simulink library "library"  (R2023b)
settings: Solver=VariableStepAuto  StartTime=0.0  StopTime=10.0  RelTol=1e-3
undefined symbols (not defined in the file or in its folder): DiscIntNeverNeededParam, mmc
libraries: $bdroot x3, spsVoltageMeasurementLib x3, spsControlledVoltageSourceLib x3, eeDiscretePi x2, spsFullBridgeMMCLib x1, simulink x1
settings Model: Creator=ma1155716  LastModifiedBy=ma1155716

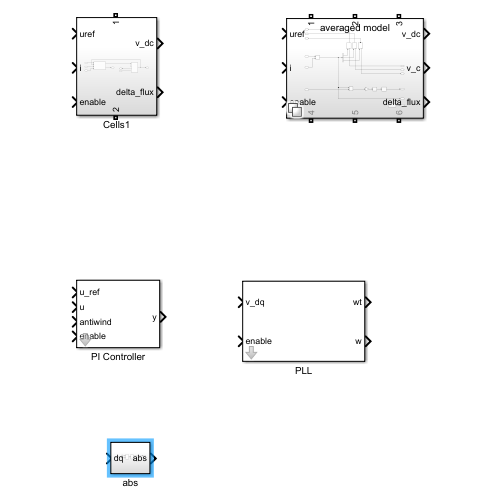
[thumbnail: Simulink's stored preview of the top-level diagram]
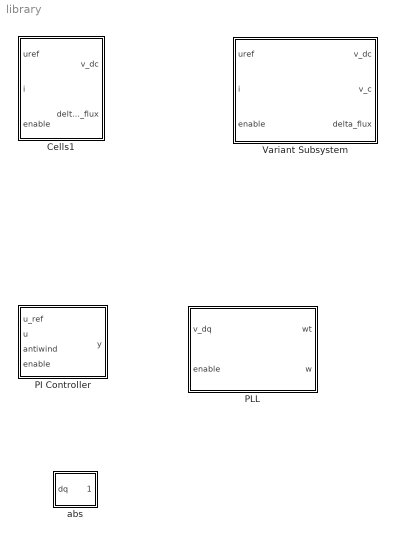
== system library ==
  Cells1 : Subsystem
      settings: PortSchema="{\"entries\":[{\"content\":{\"sides\":[{\"content\":{\"connectorIds\":[\"In1\",\"In2\",\"In3\"]},\"type\":\"ConnectorPlacement.EquallySpacedRectSide\",\"uuid\":\"5601622e-70e0-44e7-973e-d59d180f15ed\"},{\"content\":{\"connectorIds\":[\"Out1\",\"Out2\"],\"side\":\"RIGHT\"},\"type\":\"ConnectorPlacement.EquallySpacedRectSide\",\"uuid\":\"4beaff91-e32f-480b-a73b-58099df36fbd\"},{\"content\":{\"connectorIds\":[\"LConn1\"],\"side\":\"TOP\"},\"type\":\"ConnectorPlacement.EquallySpacedRectSide\",\"uuid\":\"32571f3d-d835-4e58-b20d-9f53f86bf78d\"},{\"content\":{\"connectorIds\":[\"RConn1\"],\"side\":\"BOTTOM\"},\"type\":\"ConnectorPlacement.EquallySpacedRectSide\",\"uuid\":\"b1b232fc-3b26-4ea5-8985-03b3a1c4d3e8\"}]},\"type\":\"ConnectorPlacement.EquallySpacedConnector\",\"uuid\":\"974b71ee-efdc-4c08-8e6f-7a03276fde15\"}],\"packageUris\":[\"http://schema.mathworks.com/mf0/Connector/R2020b\"],\"version\":\"1.0\"}"
  PI Controller : Subsystem  VariantControl=overcurr_ctrl.sel==1  mask{kp=0, ti=0, Kaw=1}
      mask prompts: kp "Proportional gain"; ti "Time constant"; Kaw "Anti windup gain"
  PLL : Subsystem  mask{kp=0, ti=0, w0=0, wn=0}
      mask prompts: kp "Proportional gain"; ti "Time constant"; w0 "Initial angular frequency"; wn "Nominal angular frequency"
  Variant Subsystem : Subsystem  Variant=on
      settings: PortSchema="{\"entries\":[{\"content\":{\"sides\":[{\"content\":{\"connectorIds\":[\"In1\",\"In2\",\"In3\"]},\"type\":\"ConnectorPlacement.EquallySpacedRectSide\",\"uuid\":\"07cc1b48-4eec-48c8-b7e1-ba85327af049\"},{\"content\":{\"connectorIds\":[\"Out1\",\"Out2\",\"Out3\"],\"side\":\"RIGHT\"},\"type\":\"ConnectorPlacement.EquallySpacedRectSide\",\"uuid\":\"e630ccd2-bced-4562-b965-5ba67d1cb520\"},{\"content\":{\"connectorIds\":[\"LConn1\",\"LConn2\",\"LConn3\"],\"side\":\"TOP\"},\"type\":\"ConnectorPlacement.EquallySpacedRectSide\",\"uuid\":\"f7ee33a5-0b9e-482c-ae72-b6ca50f6d328\"},{\"content\":{\"connectorIds\":[\"RConn1\",\"RConn2\",\"RConn3\"],\"side\":\"BOTTOM\"},\"type\":\"ConnectorPlacement.EquallySpacedRectSide\",\"uuid\":\"76c11136-f7c0-446b-9aed-353e2cf8a045\"}]},\"type\":\"ConnectorPlacement.EquallySpacedConnector\",\"uuid\":\"ad2af07b-650a-4f66-848d-c3c749fafa1e\"}],\"packageUris\":[\"http://schema.mathworks.com/mf0/Connector/R2020b\"],\"version\":\"1.0\"}"
  abs : Subsystem

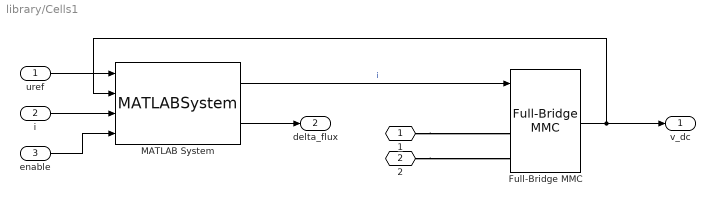
== system library/Cells1 ==
  uref : Inport
  i : Inport  Port=2
  enable : Inport  Port=3
  Full-Bridge MMC : spsFullBridgeMMCLib/Full-Bridge MMC  ModelType=Switching devices  n=mmc.cell.n  C=mmc.cell.c_dc  Vc_Initial=mmc.cell.v_dc  Ron=1e-3  Rs=1e6  Cs=inf  Ron_Diode=1e-3  Rs_Diode=1e6  Cs_Diode=inf  Vf_Diode=1e-3  Rs_CurrentSource=inf  Ts=10e-6
      settings: LibrarySourceBlock=sps_lib/Power Electronics/Full-Bridge MMC
  MATLAB System : MATLABSystem  System=CellSelector  ts=[1e-6]  f_carr=[3*50]  n_cells=[mmc.cell.n]  SimulateUsing=Code generation
      mask Type: CellSelector
      mask Display:
      | disp('CellSelector');
      | port_label('input',1,'v_ref');
      | port_label('input',2,'v_dc');
      | port_label('input',3,'i');
      | port_label('input',4,'enable');
      | port_label('output',1,'g');
      | port_label('output',2,'delta_flux');
  1 : PMIOPort  Side=Left
  2 : PMIOPort  Port=2  Side=Right
  v_dc : Outport
  delta_flux : Outport  Port=2
  wires:
  i/1 -> MATLAB System/3
  MATLAB System/2 -> delta_flux/1
  MATLAB System/1 -> Full-Bridge MMC/1  "i"
  uref/1 -> MATLAB System/1
  Full-Bridge MMC/1 -> MATLAB System/2, v_dc/1
  enable/1 -> MATLAB System/4
  connections:
  1/RConn1 -- Full-Bridge MMC/LConn1
  2/RConn1 -- Full-Bridge MMC/LConn2

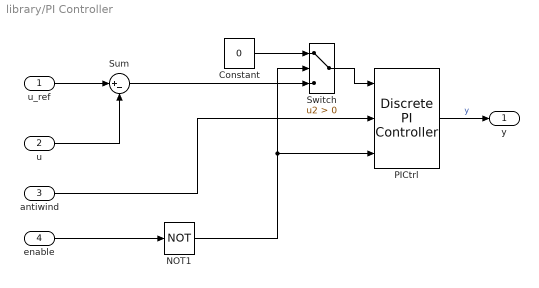
== system library/PI Controller ==
  u_ref : Inport
  u : Inport  Port=2
  antiwind : Inport  Port=3
  enable : Inport  Port=4
  Constant : Constant  Value=0
  NOT1 : Logic  Operator=NOT  IconShape=distinctive  AllPortsSameDT=off  OutDataTypeStr=boolean
  PICtrl : eeDiscretePi/Discrete PI Controller  Kp=kp  Ki=kp/ti  Kaw=Kaw  x0=0  Ts=-1
      settings: LibrarySourceBlock=ee_sl_lib/General Control/Discrete PI Controller
  Sum : Sum  Inputs=|+-
  Switch : Switch  Criteria=u2 > Threshold  SaturateOnIntegerOverflow=off  InputSameDT=off
  y : Outport
  wires:
  u_ref/1 -> Sum/1
  u/1 -> Sum/2
  NOT1/1 -> Switch/2, PICtrl/3
  enable/1 -> NOT1/1
  PICtrl/1 -> y/1  "y"
  antiwind/1 -> PICtrl/2
  Constant/1 -> Switch/1
  Switch/1 -> PICtrl/1
  Sum/1 -> Switch/3

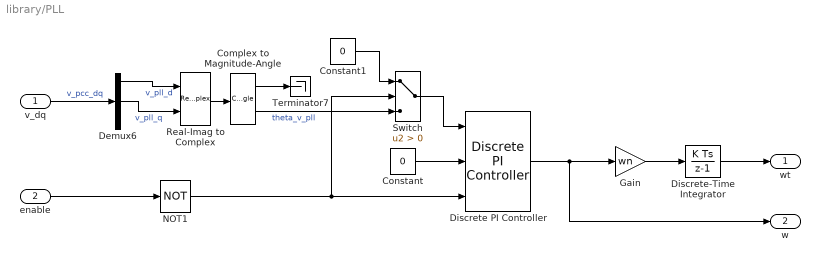
== system library/PLL ==
  v_dq : Inport
  enable : Inport  Port=2
  Complex to Magnitude-Angle : ComplexToMagnitudeAngle
  Constant : Constant  Value=0
  Constant1 : Constant  Value=0
  Demux6 : Demux  Outputs=3
  Discrete PI Controller : eeDiscretePi/Discrete PI Controller  Kp=kp  Ki=ti  Kaw=1  x0=w0  Ts=-1
      settings: LibrarySourceBlock=ee_sl_lib/General Control/Discrete PI Controller
  Discrete-Time Integrator : DiscreteIntegrator  gainval=1  SampleTime=-1  ICPrevOutput=DiscIntNeverNeededParam  ICPrevScaledInput=DiscIntNeverNeededParam
  Gain : Gain  Gain=wn
  NOT1 : Logic  Operator=NOT  IconShape=distinctive  AllPortsSameDT=off  OutDataTypeStr=boolean
  Real-Imag to Complex : RealImagToComplex
  Switch : Switch  Criteria=u2 > Threshold  SaturateOnIntegerOverflow=off  InputSameDT=off
  Terminator7 : Terminator
  wt : Outport
  w : Outport  Port=2
  wires:
  v_dq/1 -> Demux6/1  "v_pcc_dq"
  Complex to Magnitude-Angle/1 -> Terminator7/1
  Demux6/2 -> Real-Imag to Complex/2  "v_pll_q"
  Complex to Magnitude-Angle/2 -> Switch/3  "theta_v_pll"
  Real-Imag to Complex/1 -> Complex to Magnitude-Angle/1
  Demux6/1 -> Real-Imag to Complex/1  "v_pll_d"
  Constant/1 -> Discrete PI Controller/2
  Discrete PI Controller/1 -> w/1, Gain/1
  Discrete-Time Integrator/1 -> wt/1
  NOT1/1 -> Switch/2, Discrete PI Controller/3
  enable/1 -> NOT1/1
  Switch/1 -> Discrete PI Controller/1
  Constant1/1 -> Switch/1
  Gain/1 -> Discrete-Time Integrator/1

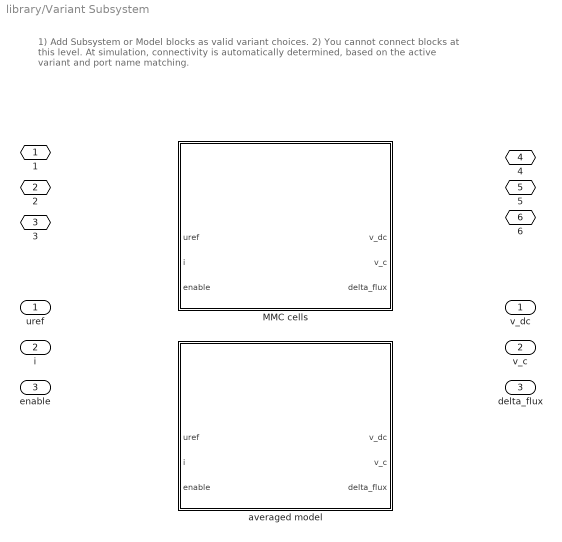
== system library/Variant Subsystem ==
  note: 1) Add Subsystem or Model blocks as valid variant choices.
      | 2) You cannot connect blocks at this level. At simulation, connectivity is automatically
      | determined, based on the active variant and port name matching.
  uref : Inport
  i : Inport  Port=2
  enable : Inport  Port=3
  MMC cells : Subsystem  VariantControl=ctrl.cell.sel==0
      settings: PortSchema="{\"entries\":[{\"content\":{\"sides\":[{\"content\":{\"connectorIds\":[\"LConn1\",\"LConn2\",\"LConn3\",\"In1\",\"In2\",\"In3\"]},\"type\":\"ConnectorPlacement.EquallySpacedRectSide\",\"uuid\":\"84231cbf-abba-4b82-bf0f-a95757b0b63e\"},{\"content\":{\"connectorIds\":[\"RConn1\",\"RConn2\",\"RConn3\",\"Out1\",\"Out2\",\"Out3\"],\"side\":\"RIGHT\"},\"type\":\"ConnectorPlacement.EquallySpacedRectSide\",\"uuid\":\"1c2b362c-b136-4319-b8b7-d737d4dfe48e\"},{\"content\":{\"side\":\"TOP\"},\"type\":\"ConnectorPlacement.EquallySpacedRectSide\",\"uuid\":\"480cfc4e-6f10-4d4d-b97c-89ec5b71d28d\"},{\"content\":{\"side\":\"BOTTOM\"},\"type\":\"ConnectorPlacement.EquallySpacedRectSide\",\"uuid\":\"2a0de7a2-5c41-412a-b00f-a11f06d7a8a4\"}]},\"type\":\"ConnectorPlacement.EquallySpacedConnector\",\"uuid\":\"a8daf21d-746a-4b9a-9b4b-aa29e4131c8e\"}],\"packageUris\":[\"http://schema.mathworks.com/mf0/Connector/R2020b\"],\"version\":\"1.0\"}"
  averaged model : Subsystem  VariantControl=ctrl.cell.sel==1
      settings: PortSchema="{\"entries\":[{\"content\":{\"sides\":[{\"content\":{\"connectorIds\":[\"LConn1\",\"LConn2\",\"LConn3\",\"In1\",\"In2\",\"In3\"]},\"type\":\"ConnectorPlacement.EquallySpacedRectSide\",\"uuid\":\"84231cbf-abba-4b82-bf0f-a95757b0b63e\"},{\"content\":{\"connectorIds\":[\"RConn1\",\"RConn2\",\"RConn3\",\"Out1\",\"Out2\",\"Out3\"],\"side\":\"RIGHT\"},\"type\":\"ConnectorPlacement.EquallySpacedRectSide\",\"uuid\":\"1c2b362c-b136-4319-b8b7-d737d4dfe48e\"},{\"content\":{\"side\":\"TOP\"},\"type\":\"ConnectorPlacement.EquallySpacedRectSide\",\"uuid\":\"480cfc4e-6f10-4d4d-b97c-89ec5b71d28d\"},{\"content\":{\"side\":\"BOTTOM\"},\"type\":\"ConnectorPlacement.EquallySpacedRectSide\",\"uuid\":\"2a0de7a2-5c41-412a-b00f-a11f06d7a8a4\"}]},\"type\":\"ConnectorPlacement.EquallySpacedConnector\",\"uuid\":\"a8daf21d-746a-4b9a-9b4b-aa29e4131c8e\"}],\"packageUris\":[\"http://schema.mathworks.com/mf0/Connector/R2020b\"],\"version\":\"1.0\"}"
  1 : PMIOPort  Side=Left
  2 : PMIOPort  Port=2  Side=Left
  3 : PMIOPort  Port=3  Side=Left
  4 : PMIOPort  Port=4  Side=Right
  5 : PMIOPort  Port=5  Side=Right
  6 : PMIOPort  Port=6  Side=Right
  v_dc : Outport
  v_c : Outport  Port=2
  delta_flux : Outport  Port=3

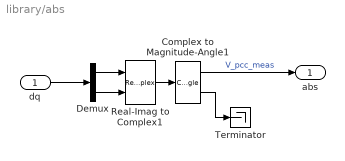
== system library/abs ==
  dq : Inport
  Complex to Magnitude-Angle1 : ComplexToMagnitudeAngle
  Demux : Demux  Outputs=2
  Real-Imag to Complex1 : RealImagToComplex
  Terminator : Terminator
  abs : Outport
  wires:
  Complex to Magnitude-Angle1/1 -> abs/1  "V_pcc_meas"
  Demux/2 -> Real-Imag to Complex1/2
  Demux/1 -> Real-Imag to Complex1/1
  Complex to Magnitude-Angle1/2 -> Terminator/1
  Real-Imag to Complex1/1 -> Complex to Magnitude-Angle1/1
  dq/1 -> Demux/1

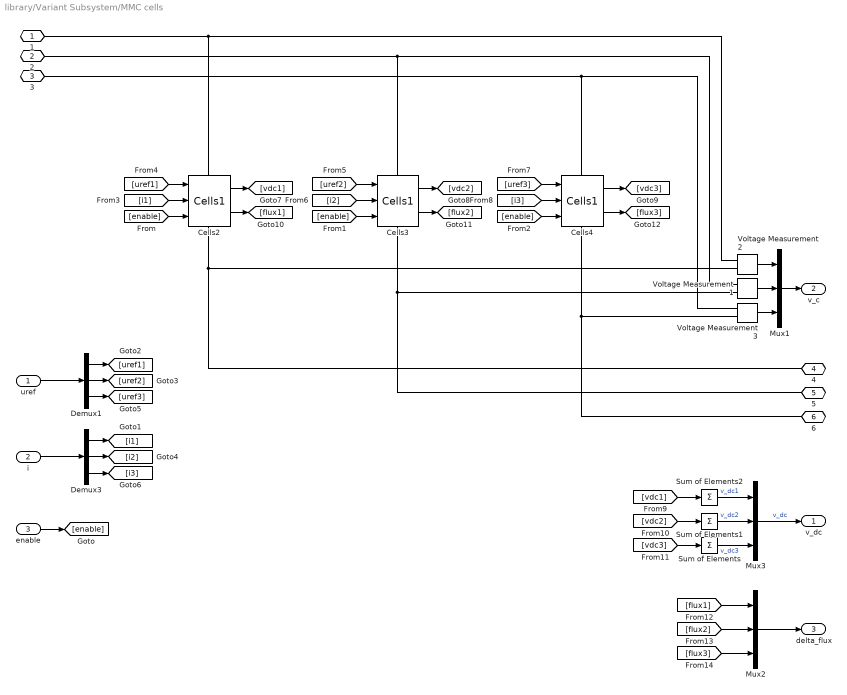
== system library/Variant Subsystem/MMC cells ==
  uref : Inport
  i : Inport  Port=2
  enable : Inport  Port=3
  Cells2 : $bdroot/Cells1  SystemSampleTime=-1  VariantActivationTime=update diagram  AllowFlexibleInterface=on  Latency=0  AutoFrameSizeCalculation=off
      settings: PortSchema="{\"entries\":[{\"content\":{\"sides\":[{\"content\":{\"connectorIds\":[\"In1\",\"In2\",\"In3\"]},\"type\":\"ConnectorPlacement.EquallySpacedRectSide\",\"uuid\":\"5601622e-70e0-44e7-973e-d59d180f15ed\"},{\"content\":{\"connectorIds\":[\"Out1\",\"Out2\"],\"side\":\"RIGHT\"},\"type\":\"ConnectorPlacement.EquallySpacedRectSide\",\"uuid\":\"4beaff91-e32f-480b-a73b-58099df36fbd\"},{\"content\":{\"connectorIds\":[\"LConn1\"],\"side\":\"TOP\"},\"type\":\"ConnectorPlacement.EquallySpacedRectSide\",\"uuid\":\"32571f3d-d835-4e58-b20d-9f53f86bf78d\"},{\"content\":{\"connectorIds\":[\"RConn1\"],\"side\":\"BOTTOM\"},\"type\":\"ConnectorPlacement.EquallySpacedRectSide\",\"uuid\":\"b1b232fc-3b26-4ea5-8985-03b3a1c4d3e8\"}]},\"type\":\"ConnectorPlacement.EquallySpacedConnector\",\"uuid\":\"974b71ee-efdc-4c08-8e6f-7a03276fde15\"}],\"packageUris\":[\"http://schema.mathworks.com/mf0/Connector/R2020b\"],\"version\":\"1.0\"}"
  Cells3 : $bdroot/Cells1  SystemSampleTime=-1  VariantActivationTime=update diagram  AllowFlexibleInterface=on  Latency=0  AutoFrameSizeCalculation=off
      settings: PortSchema="{\"entries\":[{\"content\":{\"sides\":[{\"content\":{\"connectorIds\":[\"In1\",\"In2\",\"In3\"]},\"type\":\"ConnectorPlacement.EquallySpacedRectSide\",\"uuid\":\"5601622e-70e0-44e7-973e-d59d180f15ed\"},{\"content\":{\"connectorIds\":[\"Out1\",\"Out2\"],\"side\":\"RIGHT\"},\"type\":\"ConnectorPlacement.EquallySpacedRectSide\",\"uuid\":\"4beaff91-e32f-480b-a73b-58099df36fbd\"},{\"content\":{\"connectorIds\":[\"LConn1\"],\"side\":\"TOP\"},\"type\":\"ConnectorPlacement.EquallySpacedRectSide\",\"uuid\":\"32571f3d-d835-4e58-b20d-9f53f86bf78d\"},{\"content\":{\"connectorIds\":[\"RConn1\"],\"side\":\"BOTTOM\"},\"type\":\"ConnectorPlacement.EquallySpacedRectSide\",\"uuid\":\"b1b232fc-3b26-4ea5-8985-03b3a1c4d3e8\"}]},\"type\":\"ConnectorPlacement.EquallySpacedConnector\",\"uuid\":\"974b71ee-efdc-4c08-8e6f-7a03276fde15\"}],\"packageUris\":[\"http://schema.mathworks.com/mf0/Connector/R2020b\"],\"version\":\"1.0\"}"
  Cells4 : $bdroot/Cells1  SystemSampleTime=-1  VariantActivationTime=update diagram  AllowFlexibleInterface=on  Latency=0  AutoFrameSizeCalculation=off
      settings: PortSchema="{\"entries\":[{\"content\":{\"sides\":[{\"content\":{\"connectorIds\":[\"In1\",\"In2\",\"In3\"]},\"type\":\"ConnectorPlacement.EquallySpacedRectSide\",\"uuid\":\"5601622e-70e0-44e7-973e-d59d180f15ed\"},{\"content\":{\"connectorIds\":[\"Out1\",\"Out2\"],\"side\":\"RIGHT\"},\"type\":\"ConnectorPlacement.EquallySpacedRectSide\",\"uuid\":\"4beaff91-e32f-480b-a73b-58099df36fbd\"},{\"content\":{\"connectorIds\":[\"LConn1\"],\"side\":\"TOP\"},\"type\":\"ConnectorPlacement.EquallySpacedRectSide\",\"uuid\":\"32571f3d-d835-4e58-b20d-9f53f86bf78d\"},{\"content\":{\"connectorIds\":[\"RConn1\"],\"side\":\"BOTTOM\"},\"type\":\"ConnectorPlacement.EquallySpacedRectSide\",\"uuid\":\"b1b232fc-3b26-4ea5-8985-03b3a1c4d3e8\"}]},\"type\":\"ConnectorPlacement.EquallySpacedConnector\",\"uuid\":\"974b71ee-efdc-4c08-8e6f-7a03276fde15\"}],\"packageUris\":[\"http://schema.mathworks.com/mf0/Connector/R2020b\"],\"version\":\"1.0\"}"
  Demux1 : Demux  Outputs=3
  Demux3 : Demux  Outputs=3
  Mux1 : Mux  Inputs=3
  Mux2 : Mux  Inputs=3
  Mux3 : Mux  Inputs=3
  Sum of Elements : Sum  Inputs=+
  Sum of Elements1 : Sum  Inputs=+
  Sum of Elements2 : Sum  Inputs=+
  Voltage Measurement1 : spsVoltageMeasurementLib/Voltage Measurement  PhasorSimulation=off  OutputType=Complex  PSBequivalent=0
  Voltage Measurement2 : spsVoltageMeasurementLib/Voltage Measurement  PhasorSimulation=off  OutputType=Complex  PSBequivalent=0
  Voltage Measurement3 : spsVoltageMeasurementLib/Voltage Measurement  PhasorSimulation=off  OutputType=Complex  PSBequivalent=0
  1 : PMIOPort  Side=Left
  2 : PMIOPort  Port=2  Side=Left
  3 : PMIOPort  Port=3  Side=Left
  4 : PMIOPort  Port=4  Side=Right
  5 : PMIOPort  Port=5  Side=Right
  6 : PMIOPort  Port=6  Side=Right
  v_dc : Outport
  v_c : Outport  Port=2
  delta_flux : Outport  Port=3
  wires:
  Sum of Elements1/1 -> Mux3/2  "v_dc2"
  Cells4/2 -> [flux3]
  i/1 -> Demux3/1
  Mux3/1 -> v_dc/1  "v_dc"
  Sum of Elements/1 -> Mux3/3  "v_dc3"
  Cells2/2 -> [flux1]
  Sum of Elements2/1 -> Mux3/1  "v_dc1"
  Cells3/2 -> [flux2]
  Voltage Measurement2/1 -> Mux1/1
  Voltage Measurement1/1 -> Mux1/2
  Voltage Measurement3/1 -> Mux1/3
  Mux1/1 -> v_c/1
  uref/1 -> Demux1/1
  enable/1 -> [enable]
  [enable] -> Cells2/3
  [enable] -> Cells3/3
  [enable] -> Cells4/3
  Demux3/1 -> [i1]
  [i1] -> Cells2/2
  Demux1/1 -> [uref1]
  Demux1/2 -> [uref2]
  [uref1] -> Cells2/1
  [uref2] -> Cells3/1
  Demux3/2 -> [i2]
  [i2] -> Cells3/2
  Demux1/3 -> [uref3]
  Demux3/3 -> [i3]
  [uref3] -> Cells4/1
  [i3] -> Cells4/2
  Cells2/1 -> [vdc1]
  [vdc1] -> Sum of Elements2/1
  Cells3/1 -> [vdc2]
  Cells4/1 -> [vdc3]
  [vdc2] -> Sum of Elements1/1
  [vdc3] -> Sum of Elements/1
  Mux2/1 -> delta_flux/1
  [flux1] -> Mux2/1
  [flux3] -> Mux2/3
  [flux2] -> Mux2/2
  connections:
  Cells4/RConn1 -- 6/RConn1 -- Voltage Measurement3/LConn2
  Cells4/LConn1 -- Voltage Measurement3/LConn1 -- 3/RConn1
  Cells3/RConn1 -- 5/RConn1 -- Voltage Measurement1/LConn2
  Voltage Measurement1/LConn1 -- Cells3/LConn1 -- 2/RConn1
  Voltage Measurement2/LConn1 -- Cells2/LConn1 -- 1/RConn1
  Cells2/RConn1 -- 4/RConn1 -- Voltage Measurement2/LConn2

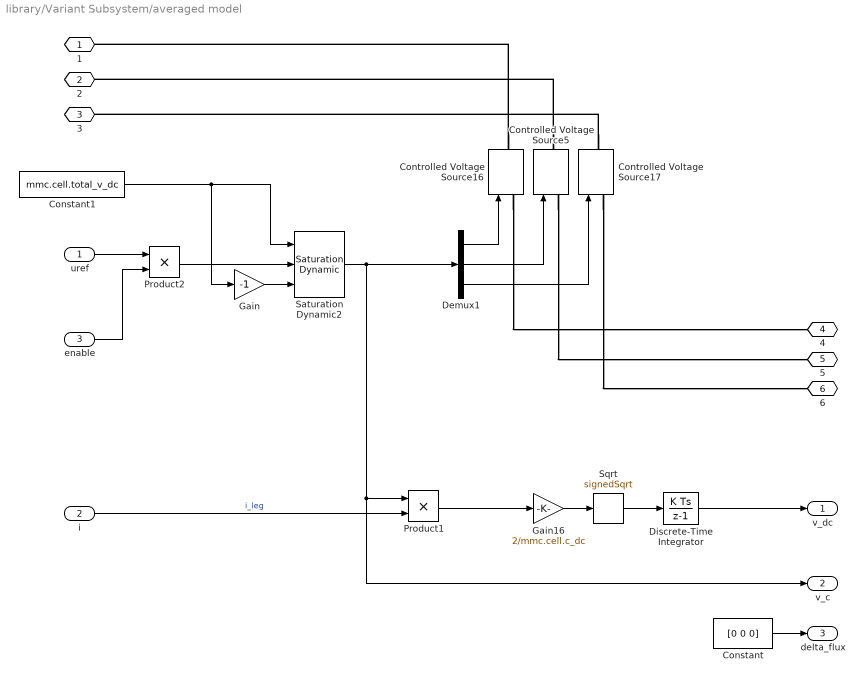
== system library/Variant Subsystem/averaged model ==
  uref : Inport
  i : Inport  Port=2
  enable : Inport  Port=3
  Constant : Constant  Value=[0 0 0]
  Constant1 : Constant  Value=mmc.cell.total_v_dc
  Controlled Voltage Source16 : spsControlledVoltageSourceLib/Controlled Voltage Source  Initialize=on  Source_Type=AC  Amplitude=0  Phase=0  Frequency=0  Measurements=None
  Controlled Voltage Source17 : spsControlledVoltageSourceLib/Controlled Voltage Source  Initialize=on  Source_Type=AC  Amplitude=0  Phase=0  Frequency=0  Measurements=None
  Controlled Voltage Source5 : spsControlledVoltageSourceLib/Controlled Voltage Source  Initialize=on  Source_Type=AC  Amplitude=0  Phase=0  Frequency=0  Measurements=None
  Demux1 : Demux  Outputs=3
  Discrete-Time Integrator : DiscreteIntegrator  gainval=1  InitialCondition=mmc.cell.v_dc*mmc.cell.n  SampleTime=-1  ICPrevOutput=DiscIntNeverNeededParam  ICPrevScaledInput=DiscIntNeverNeededParam
  Gain : Gain  Gain=-1
  Gain16 : Gain  Gain=2/mmc.cell.c_dc
  Product1 : Product
  Product2 : Product
  Saturation Dynamic2 : simulink/Discontinuities/Saturation Dynamic  OutMin=[]  OutMax=[]  OutDataTypeStr=Inherit: Same as second input  OutDataType=fixdt(1, 16)  OutScaling=2^-10  DoSatur=off
  Sqrt : Sqrt  Operator=signedSqrt
  1 : PMIOPort  Side=Left
  2 : PMIOPort  Port=2  Side=Left
  3 : PMIOPort  Port=3  Side=Left
  4 : PMIOPort  Port=4  Side=Right
  5 : PMIOPort  Port=5  Side=Right
  6 : PMIOPort  Port=6  Side=Right
  v_dc : Outport
  v_c : Outport  Port=2
  delta_flux : Outport  Port=3
  wires:
  enable/1 -> Product2/2
  Saturation Dynamic2/1 -> v_c/1, Product1/1, Demux1/1
  Sqrt/1 -> Discrete-Time Integrator/1
  Product1/1 -> Gain16/1
  Demux1/3 -> Controlled Voltage Source17/1
  i/1 -> Product1/2  "i_leg"
  Demux1/1 -> Controlled Voltage Source16/1
  Gain16/1 -> Sqrt/1
  Demux1/2 -> Controlled Voltage Source5/1
  uref/1 -> Product2/1
  Discrete-Time Integrator/1 -> v_dc/1
  Constant/1 -> delta_flux/1
  Product2/1 -> Saturation Dynamic2/2
  Constant1/1 -> Gain/1, Saturation Dynamic2/1
  Gain/1 -> Saturation Dynamic2/3
  connections:
  Controlled Voltage Source16/LConn1 -- 4/RConn1
  Controlled Voltage Source5/LConn1 -- 5/RConn1
  Controlled Voltage Source17/LConn1 -- 6/RConn1
  Controlled Voltage Source17/RConn1 -- 3/RConn1
  Controlled Voltage Source16/RConn1 -- 1/RConn1
  Controlled Voltage Source5/RConn1 -- 2/RConn1
